simulink model "OverCurrentRelay"  (R2018a)
settings: Solver=VariableStepAuto  StartTime=0.0  StopTime=0.3  RelTol=1e-3
libraries: powerlib x6, powerlib_meascontrol x3, simulink_extras x3
settings Model: Creator=Bhaskar  LastModifiedBy=Bhaskar

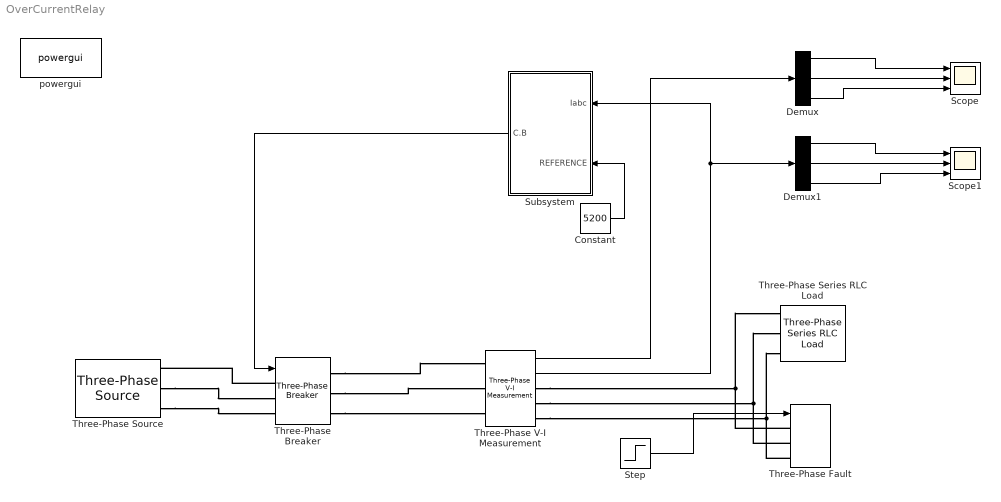
== system OverCurrentRelay ==
  Constant : Constant  Value=5200  OutDataTypeStr=boolean
  Demux : Demux  Outputs=3
  Demux1 : Demux  Outputs=3
  Scope : Scope  NumInputPorts=3
  Scope1 : Scope  NumInputPorts=3
  Step : Step  Time=0.16  Before=1  After=0  SampleTime=0
  Subsystem : Subsystem
  Three-Phase Series RLC Load : powerlib/Elements/Three-Phase Series RLC Load  LConnTagsString=A|B|C  Configuration=Y (grounded)  NominalVoltage=11e3  Vabc=[1e3 1e3 1e3]  Vabcp=[1e3 1e3 1e3]  NominalFrequency=50  UnbalancedPower=off  ActivePower=200e6  InductivePower=100  CapacitivePower=0  Pabc=[10e3 9e3 11e3]  QLabc=[100 90 110]  QCabc=[100 90 110]  Pabcp=[10e3 9e3 11e3]  QLabcp=[100 90 110]  QCabcp=[100 90 110]  Measurements=None  LoadType=constant Z
  Three-Phase V-I Measurement : powerlib/Measurements/Three-Phase V-I Measurement  VoltageMeasurement=phase-to-ground  SetLabelV=off  LabelV=Vabc  Vpu=off  VpuLL=off  CurrentMeasurement=yes  SetLabelI=off  LabelI=Iabc  Ipu=off  Pbase=100e6  Vbase=500e3  OutputType=Complex  PhasorSimulation=off  PSBequivalent=0
  Three-Phase Breaker : powerlib/Elements/Three-Phase Breaker  InitialState=closed  SwitchA=on  SwitchB=on  SwitchC=on  SwitchTimes="[1/60  5/60]"  External=on  BreakerResistance=0.001  SnubberResistance=1e6  SnubberCapacitance=inf  Measurements=None
  Three-Phase Fault : powerlib/Elements/Three-Phase Fault  InitialStates=[0 0 0]  FaultA=on  FaultB=on  FaultC=on  GroundFault=on  SwitchTimes="[1/60  5/60]"  External=on  SwitchStatus=NaN  FaultResistance=0.001  GroundResistance=0.01  SnubberResistance=1e6  SnubberCapacitance=inf  Measurements=None
  Three-Phase Source : powerlib/Electrical Sources/Three-Phase Source  InternalConnection=Yg  VoltagePhases=off  Voltage=11e3  PhaseAngle=0  Voltage_phases=[25e3 25e3 25e3]/sqrt(3)  PhaseAngles_phases=[0 -120 +120]  Frequency=50  NonIdealSource=on  SpecifyImpedance=on  Resistance=0.8929  Inductance=16.58e-3  ShortCircuitLevel=100e6  BaseVoltage=25e3  XRratio=7  BusType=swing  Pref=10e3  Qref=0  Prefabc=[10e3, 10e3, 10e3]  Qrefabc=[0, 0, 0]  Qmin=-inf  Qmax=inf
  powergui : powerlib/powergui  Priority=1  SimulationMode=Continuous  SampleTime=50e-6  frequency=60  Iterations=50  frequencyindice=50  Pbase=100e6  ErrMax=1e-4  UnitsV=kV  UnitsW=MW  buscounter=0  FunctionMessages=off  echomessages=off  EnableUseOfTLC=off  CurrentSourceSwitches=off  DisableSnubberDevices=off  DisableRonSwitches=off  DisableVfSwitches=off  DisplayEquations=off  SolverType=Tustin/Backward Euler (TBE)  Interpol=off  ExternalGateDelay=off  methode=off  Ts=100  x0status=blocks  SPID=on  SwTol=0  HookPort=off  RestoreLinks=warning  ResistiveCurrentMeasurement=off  Frange=[0:2:500]  Ylog=off  Xlog=on  ShowGrid=off  save=off  variable=ZData  structure=0  ZoomFFT=off  StartTime=0.0  cycles=1  DisplayStyle=1  fundamental=60  FreqAxis=off  MaxFrequency=1000  frequencyindicesteady=1  RmsSteady=1  display=off
  wires:
  Three-Phase V-I Measurement/2 -> Demux1/1, Subsystem/1(Iabc)
  Demux/1 -> Scope/1
  Demux/2 -> Scope/2
  Demux/3 -> Scope/3
  Demux1/2 -> Scope1/2
  Demux1/1 -> Scope1/1
  Demux1/3 -> Scope1/3
  Three-Phase V-I Measurement/1 -> Demux/1
  Subsystem/1(C.B) -> Three-Phase Breaker/1
  Step/1 -> Three-Phase Fault/1
  Constant/1 -> Subsystem/2("REFERENCE ")
  connections:
  Three-Phase Breaker/LConn1 -- Three-Phase Source/RConn1
  Three-Phase Source/RConn2 -- Three-Phase Breaker/LConn2
  Three-Phase Source/RConn3 -- Three-Phase Breaker/LConn3
  Three-Phase Breaker/RConn1 -- Three-Phase V-I Measurement/LConn1
  Three-Phase Breaker/RConn2 -- Three-Phase V-I Measurement/LConn2
  Three-Phase Breaker/RConn3 -- Three-Phase V-I Measurement/LConn3
  Three-Phase Fault/LConn1 -- Three-Phase Series RLC Load/LConn1 -- Three-Phase V-I Measurement/RConn1
  Three-Phase Fault/LConn2 -- Three-Phase Series RLC Load/LConn2 -- Three-Phase V-I Measurement/RConn2
  Three-Phase Fault/LConn3 -- Three-Phase Series RLC Load/LConn3 -- Three-Phase V-I Measurement/RConn3

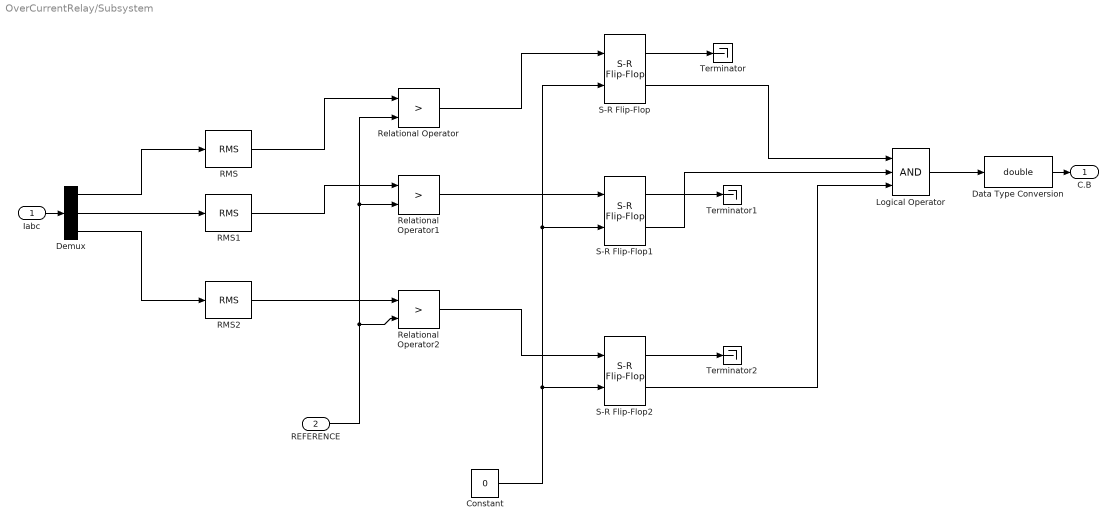
== system OverCurrentRelay/Subsystem ==
  Iabc : Inport
  "REFERENCE " : Inport  Port=2  OutDataTypeStr=boolean
  Constant : Constant  Value=0  OutDataTypeStr=boolean
  Data Type Conversion : DataTypeConversion  OutDataTypeStr=double
  Demux : Demux  Outputs=3
  Logical Operator : Logic  Inputs=3  AllPortsSameDT=off  OutDataTypeStr=boolean
  RMS : powerlib_meascontrol/Measurements/RMS  TrueRMS=on  Freq=50  RMSInit=120  Ts=0
  RMS1 : powerlib_meascontrol/Measurements/RMS  TrueRMS=on  Freq=50  RMSInit=120  Ts=0
  RMS2 : powerlib_meascontrol/Measurements/RMS  TrueRMS=on  Freq=50  RMSInit=120  Ts=0
  Relational Operator : RelationalOperator  Operator=>  OutDataTypeStr=boolean  RndMeth=Simplest
  Relational Operator1 : RelationalOperator  Operator=>  OutDataTypeStr=boolean  RndMeth=Simplest
  Relational Operator2 : RelationalOperator  Operator=>  OutDataTypeStr=boolean  RndMeth=Simplest
  S-R Flip-Flop : simulink_extras/Flip Flops/S-R Flip-Flop  initial_condition=0
  S-R Flip-Flop1 : simulink_extras/Flip Flops/S-R Flip-Flop  initial_condition=0
  S-R Flip-Flop2 : simulink_extras/Flip Flops/S-R Flip-Flop  initial_condition=0
  Terminator : Terminator
  Terminator1 : Terminator
  Terminator2 : Terminator
  C.B : Outport
  wires:
  RMS1/1 -> Relational Operator1/1
  Demux/2 -> RMS1/1
  RMS/1 -> Relational Operator/1
  Relational Operator2/1 -> S-R Flip-Flop2/1
  S-R Flip-Flop/2 -> Logical Operator/1
  Logical Operator/1 -> Data Type Conversion/1
  S-R Flip-Flop1/1 -> Terminator1/1
  Constant/1 -> S-R Flip-Flop2/2, S-R Flip-Flop1/2, S-R Flip-Flop/2
  S-R Flip-Flop/1 -> Terminator/1
  "REFERENCE "/1 -> Relational Operator2/2, Relational Operator1/2, Relational Operator/2
  Demux/3 -> RMS2/1
  Demux/1 -> RMS/1
  S-R Flip-Flop2/2 -> Logical Operator/3
  Relational Operator/1 -> S-R Flip-Flop/1
  RMS2/1 -> Relational Operator2/1
  Data Type Conversion/1 -> C.B/1
  S-R Flip-Flop2/1 -> Terminator2/1
  S-R Flip-Flop1/2 -> Logical Operator/2
  Relational Operator1/1 -> S-R Flip-Flop1/1
  Iabc/1 -> Demux/1
